simulink model "Detector1"  (R2017b)
settings: Solver=ode3  StartTime=0.0  StopTime=10.0  FixedStep=0.200000  RelTol=1e-3
libraries: sldvlib x8
settings Model: Creator=hbourbou  LastModifiedBy=hbourbou
settings OptimizationCC: LifeSpan=inf
settings DebuggingCC: SFExecutionAtInitializationDiag=none
settings HardwareCC: ProdBitPerSizeT=32  ProdBitPerPtrDiffT=32  ProdWordSize=32  ProdHWDeviceType=Specified
settings CodeAppCC: StateflowObjectComments=on

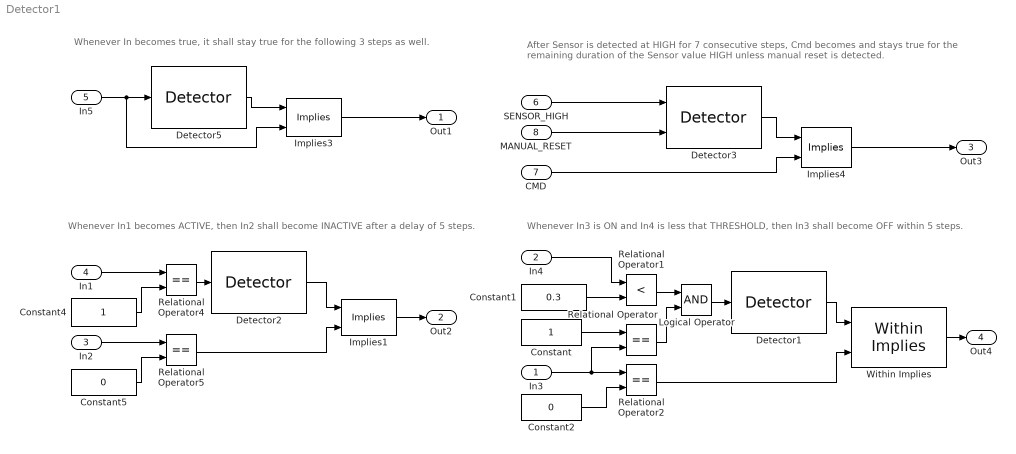
== system Detector1 ==
  note: After Sensor is detected at HIGH for 7 consecutive steps, Cmd becomes and stays true for
      | the remaining duration of the Sensor value HIGH unless manual reset is detected.
  note: Whenever In3 is ON and In4 is less that THRESHOLD, then In3 shall become OFF within 5 steps.
  note: Whenever In becomes true, it shall stay true for the following 3 steps as well.
  note: Whenever In1 becomes ACTIVE, then In2 shall become INACTIVE after a delay of 5 steps.
  In3 : Inport  OutDataTypeStr=boolean
  In4 : Inport  Port=2
  In2 : Inport  Port=3
  In1 : Inport  Port=4
  In5 : Inport  Port=5  OutDataTypeStr=boolean
  SENSOR_HIGH : Inport  Port=6
  CMD : Inport  Port=7
  MANUAL_RESET : Inport  Port=8  OutDataTypeStr=boolean
  Constant : Constant
  Constant1 : Constant  Value=0.3
  Constant2 : Constant  Value=0
  Constant4 : Constant
  Constant5 : Constant  Value=0
  Detector1 : sldvlib/Temporal Operators/Detector  reset=off  typ=Delayed Fixed Duration  in_hold=1  delay=0  out_hold=5
      settings: SourceProductName=Simulink Design Verifier  SourceProductBaseCode=DV
  Detector2 : sldvlib/Temporal Operators/Detector  reset=off  typ=Delayed Fixed Duration  in_hold=1  delay=5  out_hold=1
      settings: SourceProductName=Simulink Design Verifier  SourceProductBaseCode=DV
  Detector3 : sldvlib/Temporal Operators/Detector  reset=on  typ=Synchronized  in_hold=7  delay=0  out_hold=5
      settings: SourceProductName=Simulink Design Verifier  SourceProductBaseCode=DV
  Detector5 : sldvlib/Temporal Operators/Detector  reset=off  typ=Delayed Fixed Duration  in_hold=1  delay=2  out_hold=3
      settings: SourceProductName=Simulink Design Verifier  SourceProductBaseCode=DV
  Implies1 : sldvlib/Verification Utilities/Implies
      settings: SourceProductName=Simulink Design Verifier  SourceProductBaseCode=DV
  Implies3 : sldvlib/Verification Utilities/Implies
      settings: SourceProductName=Simulink Design Verifier  SourceProductBaseCode=DV
  Implies4 : sldvlib/Verification Utilities/Implies
      settings: SourceProductName=Simulink Design Verifier  SourceProductBaseCode=DV
  Logical Operator : Logic  AllPortsSameDT=off  OutDataTypeStr=boolean
  Relational Operator{,2,4..5} (4 alike) : RelationalOperator  Operator===  OutDataTypeStr=boolean  RndMeth=Nearest
  Relational Operator1 : RelationalOperator  Operator=<  OutDataTypeStr=boolean  RndMeth=Nearest
  Within Implies : sldvlib/Temporal Operators/Within Implies  reset=off
      settings: SourceProductName=Simulink Design Verifier  SourceProductBaseCode=DV
  Out1 : Outport
  Out2 : Outport  Port=2
  Out3 : Outport  Port=3
  Out4 : Outport  Port=4
  wires:
  Detector2/1 -> Implies1/1
  Detector3/1 -> Implies4/1
  Constant5/1 -> Relational Operator5/2
  Implies1/1 -> Out2/1
  Constant4/1 -> Relational Operator4/2
  Relational Operator2/1 -> Within Implies/2
  In3/1 -> Relational Operator2/1, Relational Operator/2
  In1/1 -> Relational Operator4/1
  Relational Operator1/1 -> Logical Operator/1
  Logical Operator/1 -> Detector1/1
  Within Implies/1 -> Out4/1
  In2/1 -> Relational Operator5/1
  Constant2/1 -> Relational Operator2/2
  Detector1/1 -> Within Implies/1
  Detector5/1 -> Implies3/1
  Relational Operator5/1 -> Implies1/2
  In5/1 -> Implies3/2, Detector5/1
  Relational Operator4/1 -> Detector2/1
  Constant/1 -> Relational Operator/1
  Relational Operator/1 -> Logical Operator/2
  Implies3/1 -> Out1/1
  In4/1 -> Relational Operator1/1
  Implies4/1 -> Out3/1
  SENSOR_HIGH/1 -> Detector3/1
  Constant1/1 -> Relational Operator1/2
  MANUAL_RESET/1 -> Detector3/2
  CMD/1 -> Implies4/2
